simulink library "InterModuleProtocol"  (R2020b)
settings: Solver=VariableStepAuto  StartTime=0.0  StopTime=10.0  RelTol=1e-3
(part 2 of 2)

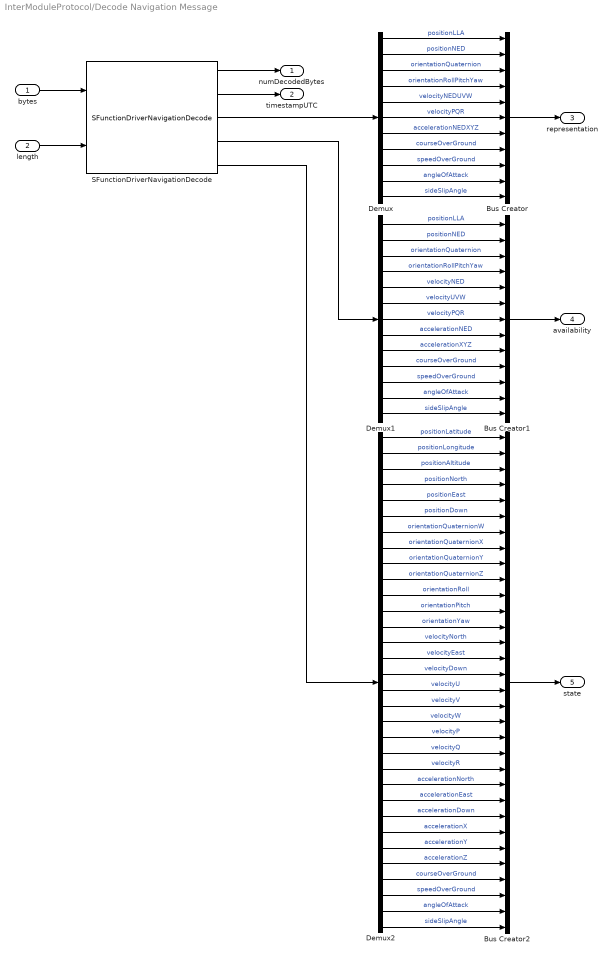
== system InterModuleProtocol/Decode Navigation Message ==
  bytes : Inport  OutDataTypeStr=uint8  PortDimensions=268
  length : Inport  Port=2  OutDataTypeStr=uint32  PortDimensions=1
  Bus Creator : BusCreator  Inputs=11
  Bus Creator1 : BusCreator  Inputs=13
  Bus Creator2 : BusCreator  Inputs=32
  Demux : Demux  Outputs=11
  Demux1 : Demux  Outputs=13
  Demux2 : Demux  Outputs=32
  SFunctionDriverNavigationDecode : S-Function  FunctionName=SFunctionDriverNavigationDecode  Parameters=SampleTime  SFunctionDeploymentMode=off  EnableBusSupport=off  mask(Legacy Function){SFunctionSpec=void OutputDriverNavigationDecode(uint8 u1[], uint32 u2, int32 y1[1], double y2[1], uint8 y3[11], uint8 y4[13], double y5[32]), SampleTime=-1, ShowSpec=off}
      mask prompts: SampleTime "Sample time (-1 for inherited):"; ShowSpec "Display function specification"
      mask help:
      | This block allows you to call the legacy functions specified by the following Legacy Code Tool definition:
      | def.SFunctionName = 'SFunctionDriverNavigationDecode';
      | def.OutputFcnSpec = 'void OutputDriverNavigationDecode(uint8 u1[], uint32 u2, int32 y1[1], double y2[1], uint8 y3[11], uint8 y4[13], double y5[32])';
      | def.StartFcnSpec = 'void CreateDriverNavigationDecode()';
      | def.TerminateFcnSpec = 'void DeleteDriverNavigationDecode()';
      | def.HeaderFiles = {'DriverNavigationDecode.h'};
      | def.SourceFiles = {'DriverNavigationDecode.cpp', 'InterModuleProtocol.cpp', 'IMPState.cpp', 'IMPStateConfiguration.cpp'};
      | def.SampleTime = 'parameterized';
      | def.Options.useTlcWithAccel = false;
      mask Help: <p>This block was generated automatically by the Legacy Code Tool. For detailed help on this tool, call<a href="matlab:legacy_code('help')"> legacy_code('help')</a>.</p>
      mask Callback ShowSpec:
      | if strcmp(get_param(gcbh, 'ShowSpec'), 'on')
      |   set_param(gcbh, 'MaskDisplay', sprintf('fprintf(''%s'');', get_param(gcbh, 'SFunctionSpec')));
      | else
      |   set_param(gcbh, 'MaskDisplay', sprintf('fprintf(''%s'');', get_param(gcbh, 'FunctionName')));
      | end
      mask Display: fprintf('SFunctionDriverNavigationDecode');
  numDecodedBytes : Outport  OutDataTypeStr=int32  PortDimensions=1  VectorParamsAs1DForOutWhenUnconnected=off
  timestampUTC : Outport  Port=2  OutDataTypeStr=double  Unit=s  PortDimensions=1  VectorParamsAs1DForOutWhenUnconnected=off
  representation : Outport  Port=3  OutDataTypeStr=uint8  PortDimensions=11  VectorParamsAs1DForOutWhenUnconnected=off
  availability : Outport  Port=4  OutDataTypeStr=uint8  PortDimensions=13  VectorParamsAs1DForOutWhenUnconnected=off
  state : Outport  Port=5  OutDataTypeStr=double  PortDimensions=32  VectorParamsAs1DForOutWhenUnconnected=off
  wires:
  SFunctionDriverNavigationDecode/1 -> numDecodedBytes/1
  SFunctionDriverNavigationDecode/2 -> timestampUTC/1
  length/1 -> SFunctionDriverNavigationDecode/2
  bytes/1 -> SFunctionDriverNavigationDecode/1
  Demux/1 -> Bus Creator/1  "positionLLA"
  Demux/2 -> Bus Creator/2  "positionNED"
  Demux/3 -> Bus Creator/3  "orientationQuaternion"
  Demux/4 -> Bus Creator/4  "orientationRollPitchYaw"
  Demux/5 -> Bus Creator/5  "velocityNEDUVW"
  Demux/6 -> Bus Creator/6  "velocityPQR"
  Demux/7 -> Bus Creator/7  "accelerationNEDXYZ"
  Demux/8 -> Bus Creator/8  "courseOverGround"
  Demux/9 -> Bus Creator/9  "speedOverGround"
  Demux/10 -> Bus Creator/10  "angleOfAttack"
  Demux/11 -> Bus Creator/11  "sideSlipAngle"
  SFunctionDriverNavigationDecode/3 -> Demux/1
  Bus Creator/1 -> representation/1
  SFunctionDriverNavigationDecode/4 -> Demux1/1
  Demux1/1 -> Bus Creator1/1  "positionLLA"
  Demux1/2 -> Bus Creator1/2  "positionNED"
  Demux1/3 -> Bus Creator1/3  "orientationQuaternion"
  Demux1/4 -> Bus Creator1/4  "orientationRollPitchYaw"
  Demux1/5 -> Bus Creator1/5  "velocityNED"
  Demux1/6 -> Bus Creator1/6  "velocityUVW"
  Demux1/7 -> Bus Creator1/7  "velocityPQR"
  Demux1/8 -> Bus Creator1/8  "accelerationNED"
  Demux1/9 -> Bus Creator1/9  "accelerationXYZ"
  Demux1/10 -> Bus Creator1/10  "courseOverGround"
  Demux1/11 -> Bus Creator1/11  "speedOverGround"
  Demux1/12 -> Bus Creator1/12  "angleOfAttack"
  Demux1/13 -> Bus Creator1/13  "sideSlipAngle"
  Bus Creator1/1 -> availability/1
  Demux2/1 -> Bus Creator2/1  "positionLatitude"
  Demux2/2 -> Bus Creator2/2  "positionLongitude"
  Demux2/3 -> Bus Creator2/3  "positionAltitude"
  Demux2/4 -> Bus Creator2/4  "positionNorth"
  Demux2/5 -> Bus Creator2/5  "positionEast"
  Demux2/6 -> Bus Creator2/6  "positionDown"
  Demux2/7 -> Bus Creator2/7  "orientationQuaternionW"
  Demux2/8 -> Bus Creator2/8  "orientationQuaternionX"
  Demux2/9 -> Bus Creator2/9  "orientationQuaternionY"
  Demux2/10 -> Bus Creator2/10  "orientationQuaternionZ"
  Demux2/11 -> Bus Creator2/11  "orientationRoll"
  Demux2/12 -> Bus Creator2/12  "orientationPitch"
  Demux2/13 -> Bus Creator2/13  "orientationYaw"
  Demux2/14 -> Bus Creator2/14  "velocityNorth"
  Demux2/15 -> Bus Creator2/15  "velocityEast"
  Demux2/16 -> Bus Creator2/16  "velocityDown"
  Demux2/17 -> Bus Creator2/17  "velocityU"
  Demux2/18 -> Bus Creator2/18  "velocityV"
  Demux2/19 -> Bus Creator2/19  "velocityW"
  Demux2/20 -> Bus Creator2/20  "velocityP"
  Demux2/21 -> Bus Creator2/21  "velocityQ"
  Demux2/22 -> Bus Creator2/22  "velocityR"
  Demux2/23 -> Bus Creator2/23  "accelerationNorth"
  Demux2/24 -> Bus Creator2/24  "accelerationEast"
  Demux2/25 -> Bus Creator2/25  "accelerationDown"
  Demux2/26 -> Bus Creator2/26  "accelerationX"
  Demux2/27 -> Bus Creator2/27  "accelerationY"
  Demux2/28 -> Bus Creator2/28  "accelerationZ"
  Demux2/29 -> Bus Creator2/29  "courseOverGround"
  Demux2/30 -> Bus Creator2/30  "speedOverGround"
  Demux2/31 -> Bus Creator2/31  "angleOfAttack"
  Demux2/32 -> Bus Creator2/32  "sideSlipAngle"
  Bus Creator2/1 -> state/1
  SFunctionDriverNavigationDecode/5 -> Demux2/1

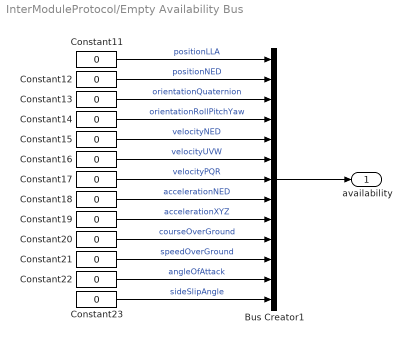
== system InterModuleProtocol/Empty Availability Bus ==
  Bus Creator1 : BusCreator  Inputs=13
  Constant{11..23} (13 alike) : Constant  Value=0  OutDataTypeStr=uint8
  availability : Outport  VectorParamsAs1DForOutWhenUnconnected=off
  wires:
  Constant21/1 -> Bus Creator1/11  "speedOverGround"
  Constant14/1 -> Bus Creator1/4  "orientationRollPitchYaw"
  Constant15/1 -> Bus Creator1/5  "velocityNED"
  Constant23/1 -> Bus Creator1/13  "sideSlipAngle"
  Bus Creator1/1 -> availability/1
  Constant12/1 -> Bus Creator1/2  "positionNED"
  Constant20/1 -> Bus Creator1/10  "courseOverGround"
  Constant16/1 -> Bus Creator1/6  "velocityUVW"
  Constant17/1 -> Bus Creator1/7  "velocityPQR"
  Constant13/1 -> Bus Creator1/3  "orientationQuaternion"
  Constant11/1 -> Bus Creator1/1  "positionLLA"
  Constant18/1 -> Bus Creator1/8  "accelerationNED"
  Constant19/1 -> Bus Creator1/9  "accelerationXYZ"
  Constant22/1 -> Bus Creator1/12  "angleOfAttack"

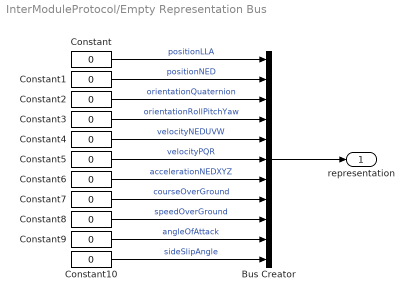
== system InterModuleProtocol/Empty Representation Bus ==
  Bus Creator : BusCreator  Inputs=11
  Constant{,1..10} (11 alike) : Constant  Value=0  OutDataTypeStr=uint8
  representation : Outport  VectorParamsAs1DForOutWhenUnconnected=off
  wires:
  Constant10/1 -> Bus Creator/11  "sideSlipAngle"
  Constant1/1 -> Bus Creator/2  "positionNED"
  Constant8/1 -> Bus Creator/9  "speedOverGround"
  Bus Creator/1 -> representation/1
  Constant9/1 -> Bus Creator/10  "angleOfAttack"
  Constant7/1 -> Bus Creator/8  "courseOverGround"
  Constant6/1 -> Bus Creator/7  "accelerationNEDXYZ"
  Constant4/1 -> Bus Creator/5  "velocityNEDUVW"
  Constant5/1 -> Bus Creator/6  "velocityPQR"
  Constant3/1 -> Bus Creator/4  "orientationRollPitchYaw"
  Constant2/1 -> Bus Creator/3  "orientationQuaternion"
  Constant/1 -> Bus Creator/1  "positionLLA"

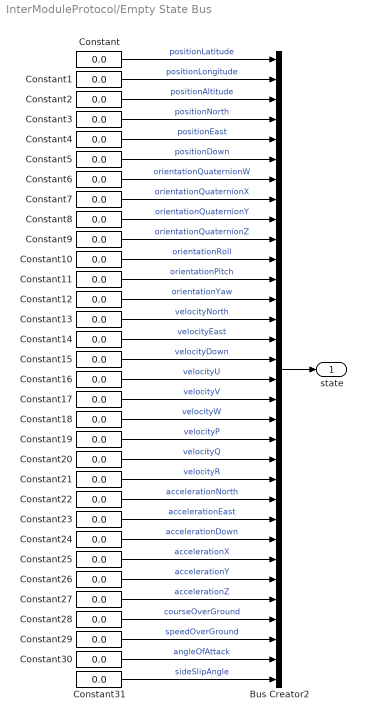
== system InterModuleProtocol/Empty State Bus ==
  Bus Creator2 : BusCreator  Inputs=32
  Constant{,1..31} (32 alike) : Constant  Value=0.0  OutDataTypeStr=double
  state : Outport  VectorParamsAs1DForOutWhenUnconnected=off
  wires:
  Constant29/1 -> Bus Creator2/30  "speedOverGround"
  Constant2/1 -> Bus Creator2/3  "positionAltitude"
  Constant8/1 -> Bus Creator2/9  "orientationQuaternionY"
  Constant17/1 -> Bus Creator2/18  "velocityV"
  Bus Creator2/1 -> state/1
  Constant25/1 -> Bus Creator2/26  "accelerationX"
  Constant1/1 -> Bus Creator2/2  "positionLongitude"
  Constant27/1 -> Bus Creator2/28  "accelerationZ"
  Constant3/1 -> Bus Creator2/4  "positionNorth"
  Constant12/1 -> Bus Creator2/13  "orientationYaw"
  Constant18/1 -> Bus Creator2/19  "velocityW"
  Constant24/1 -> Bus Creator2/25  "accelerationDown"
  Constant22/1 -> Bus Creator2/23  "accelerationNorth"
  Constant/1 -> Bus Creator2/1  "positionLatitude"
  Constant15/1 -> Bus Creator2/16  "velocityDown"
  Constant14/1 -> Bus Creator2/15  "velocityEast"
  Constant10/1 -> Bus Creator2/11  "orientationRoll"
  Constant26/1 -> Bus Creator2/27  "accelerationY"
  Constant30/1 -> Bus Creator2/31  "angleOfAttack"
  Constant6/1 -> Bus Creator2/7  "orientationQuaternionW"
  Constant13/1 -> Bus Creator2/14  "velocityNorth"
  Constant11/1 -> Bus Creator2/12  "orientationPitch"
  Constant16/1 -> Bus Creator2/17  "velocityU"
  Constant21/1 -> Bus Creator2/22  "velocityR"
  Constant19/1 -> Bus Creator2/20  "velocityP"
  Constant31/1 -> Bus Creator2/32  "sideSlipAngle"
  Constant4/1 -> Bus Creator2/5  "positionEast"
  Constant7/1 -> Bus Creator2/8  "orientationQuaternionX"
  Constant5/1 -> Bus Creator2/6  "positionDown"
  Constant9/1 -> Bus Creator2/10  "orientationQuaternionZ"
  Constant28/1 -> Bus Creator2/29  "courseOverGround"
  Constant20/1 -> Bus Creator2/21  "velocityQ"
  Constant23/1 -> Bus Creator2/24  "accelerationEast"

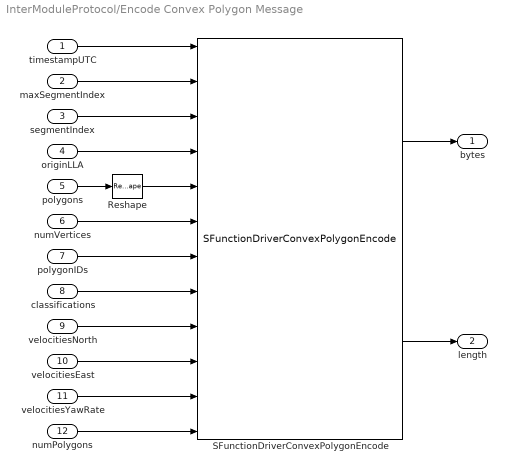
== system InterModuleProtocol/Encode Convex Polygon Message ==
  timestampUTC : Inport  OutDataTypeStr=double  Unit=s  PortDimensions=1
  maxSegmentIndex : Inport  Port=2  OutDataTypeStr=uint8  PortDimensions=1
  segmentIndex : Inport  Port=3  OutDataTypeStr=uint8  PortDimensions=1
  originLLA : Inport  Port=4  OutDataTypeStr=double  PortDimensions=3
  polygons : Inport  Port=5  OutDataTypeStr=double  Unit=m  PortDimensions=[2, 255, maxNumPolygons]
  numVertices : Inport  Port=6  OutDataTypeStr=uint8  PortDimensions=maxNumPolygons
  polygonIDs : Inport  Port=7  OutDataTypeStr=uint16  PortDimensions=maxNumPolygons
  classifications : Inport  Port=8  OutDataTypeStr=uint8  PortDimensions=maxNumPolygons
  velocitiesNorth : Inport  Port=9  OutDataTypeStr=double  Unit=m/s  PortDimensions=maxNumPolygons
  velocitiesEast : Inport  Port=10  OutDataTypeStr=double  Unit=m/s  PortDimensions=maxNumPolygons
  velocitiesYawRate : Inport  Port=11  OutDataTypeStr=double  Unit=rad/s  PortDimensions=maxNumPolygons
  numPolygons : Inport  Port=12  OutDataTypeStr=uint16  PortDimensions=1
  Reshape : Reshape  OutputDimensionality=Customize  OutputDimensions=[2*255*maxNumPolygons,1]
  SFunctionDriverConvexPolygonEncode : S-Function  FunctionName=SFunctionDriverConvexPolygonEncode  Parameters=SParameter1, SParameter2, SampleTime  SFunctionDeploymentMode=off  EnableBusSupport=off  mask(Legacy Function){SFunctionSpec=void OutputDriverConvexPolygonEncode(uint8 y1[p1], uint32 y2[1], uint32 p1, double u1, uint8 u2, uint8 u3, double u4[3], double u5[2*255*p2], uint16 p2, uint8 u6[p2], uint8 u7[p2], uint8 u8[p2], double u9[p2], double u10[p2], double u11[p2], uint16 u12), SParameter1=uint32(reshape(outBufferSize, [1 1])), SParameter2=uint16(reshape(maxNumPolygons, [1 1])), SampleTime=-1, ShowSpec=off}
      mask prompts: SParameter1 "P1:"; SParameter2 "P2:"; SampleTime "Sample time (-1 for inherited):"; ShowSpec "Display function specification"
      mask help:
      | This block allows you to call the legacy functions specified by the following Legacy Code Tool definition:
      | def.SFunctionName = 'SFunctionDriverConvexPolygonEncode';
      | def.OutputFcnSpec = 'void OutputDriverConvexPolygonEncode(uint8 y1[p1], uint32 y2[1], uint32 p1, double u1, uint8 u2, uint8 u3, double u4[3], double u5[2*255*p2], uint16 p2, uint8 u6[p2], uint8 u7[p2], uint8 u8[p2], double u9[p2], double u10[p2], double u11[p2], uint16 u12)';
      | def.StartFcnSpec = 'void CreateDriverConvexPolygonEncode()';
      | def.TerminateFcnSpec = 'void DeleteDriverConvexPolygonEncode()';
      | def.HeaderFiles = {'DriverConvexPolygonEncode.h'};
      | def.SourceFiles = {'DriverConvexPolygonEncode.cpp', 'InterModuleProtocol.cpp', 'IMPState.cpp', 'IMPConvexPolygon.cpp', 'IMPStateConfiguration.cpp'};
      | def.SampleTime = 'parameterized';
      | def.Options.useTlcWithAccel = false;
      mask Help: <p>This block was generated automatically by the Legacy Code Tool. For detailed help on this tool, call<a href="matlab:legacy_code('help')"> legacy_code('help')</a>.</p>
      mask Callback ShowSpec:
      | if strcmp(get_param(gcbh, 'ShowSpec'), 'on')
      |   set_param(gcbh, 'MaskDisplay', sprintf('fprintf(''%s'');', get_param(gcbh, 'SFunctionSpec')));
      | else
      |   set_param(gcbh, 'MaskDisplay', sprintf('fprintf(''%s'');', get_param(gcbh, 'FunctionName')));
      | end
      mask Display: fprintf('SFunctionDriverConvexPolygonEncode');
  bytes : Outport  OutDataTypeStr=uint8  PortDimensions=outBufferSize  VectorParamsAs1DForOutWhenUnconnected=off
  length : Outport  Port=2  OutDataTypeStr=uint32  PortDimensions=1  VectorParamsAs1DForOutWhenUnconnected=off
  wires:
  polygons/1 -> Reshape/1
  SFunctionDriverConvexPolygonEncode/1 -> bytes/1
  SFunctionDriverConvexPolygonEncode/2 -> length/1
  timestampUTC/1 -> SFunctionDriverConvexPolygonEncode/1
  maxSegmentIndex/1 -> SFunctionDriverConvexPolygonEncode/2
  segmentIndex/1 -> SFunctionDriverConvexPolygonEncode/3
  originLLA/1 -> SFunctionDriverConvexPolygonEncode/4
  Reshape/1 -> SFunctionDriverConvexPolygonEncode/5
  numVertices/1 -> SFunctionDriverConvexPolygonEncode/6
  polygonIDs/1 -> SFunctionDriverConvexPolygonEncode/7
  numPolygons/1 -> SFunctionDriverConvexPolygonEncode/12
  classifications/1 -> SFunctionDriverConvexPolygonEncode/8
  velocitiesNorth/1 -> SFunctionDriverConvexPolygonEncode/9
  velocitiesEast/1 -> SFunctionDriverConvexPolygonEncode/10
  velocitiesYawRate/1 -> SFunctionDriverConvexPolygonEncode/11

== system InterModuleProtocol/Encode Guidance Message ==
  timestampUTC : Inport  OutDataTypeStr=double  Unit=s  PortDimensions=1
  representation : Inport  Port=2  OutDataTypeStr=uint8  PortDimensions=11
  availability : Inport  Port=3  OutDataTypeStr=uint8  PortDimensions=13
  state : Inport  Port=4  OutDataTypeStr=double  PortDimensions=32
  SFunctionDriverGuidanceEncode : S-Function  FunctionName=SFunctionDriverGuidanceEncode  Parameters=SParameter1, SampleTime  SFunctionDeploymentMode=off  EnableBusSupport=off  mask(Legacy Function){SFunctionSpec=void OutputDriverGuidanceEncode(uint8 y1[p1], uint32 y2[1], uint32 p1, double u1, uint8 u2[11], uint8 u3[13], double u4[32]), SParameter1=uint32(reshape(outputBufferSize, [1 1])), SampleTime=-1, ShowSpec=off}
      mask prompts: SParameter1 "P1:"; SampleTime "Sample time (-1 for inherited):"; ShowSpec "Display function specification"
      mask help:
      | This block allows you to call the legacy functions specified by the following Legacy Code Tool definition:
      | def.SFunctionName = 'SFunctionDriverGuidanceEncode';
      | def.OutputFcnSpec = 'void OutputDriverGuidanceEncode(uint8 y1[p1], uint32 y2[1], uint32 p1, double u1, uint8 u2[11], uint8 u3[13], double u4[32])';
      | def.StartFcnSpec = 'void CreateDriverGuidanceEncode()';
      | def.TerminateFcnSpec = 'void DeleteDriverGuidanceEncode()';
      | def.HeaderFiles = {'DriverGuidanceEncode.h'};
      | def.SourceFiles = {'DriverGuidanceEncode.cpp', 'InterModuleProtocol.cpp', 'IMPConvexPolygon.cpp', 'IMPState.cpp', 'IMPStateConfiguration.cpp'};
      | def.SampleTime = 'parameterized';
      | def.Options.useTlcWithAccel = false;
      mask Help: <p>This block was generated automatically by the Legacy Code Tool. For detailed help on this tool, call<a href="matlab:legacy_code('help')"> legacy_code('help')</a>.</p>
      mask Callback ShowSpec:
      | if strcmp(get_param(gcbh, 'ShowSpec'), 'on')
      |   set_param(gcbh, 'MaskDisplay', sprintf('fprintf(''%s'');', get_param(gcbh, 'SFunctionSpec')));
      | else
      |   set_param(gcbh, 'MaskDisplay', sprintf('fprintf(''%s'');', get_param(gcbh, 'FunctionName')));
      | end
      mask Display: fprintf('SFunctionDriverGuidanceEncode');
  bytes : Outport  OutDataTypeStr=uint8  PortDimensions=outputBufferSize  VectorParamsAs1DForOutWhenUnconnected=off
  length : Outport  Port=2  OutDataTypeStr=uint32  PortDimensions=1  VectorParamsAs1DForOutWhenUnconnected=off
  wires:
  timestampUTC/1 -> SFunctionDriverGuidanceEncode/1
  representation/1 -> SFunctionDriverGuidanceEncode/2
  availability/1 -> SFunctionDriverGuidanceEncode/3
  state/1 -> SFunctionDriverGuidanceEncode/4
  SFunctionDriverGuidanceEncode/1 -> bytes/1
  SFunctionDriverGuidanceEncode/2 -> length/1

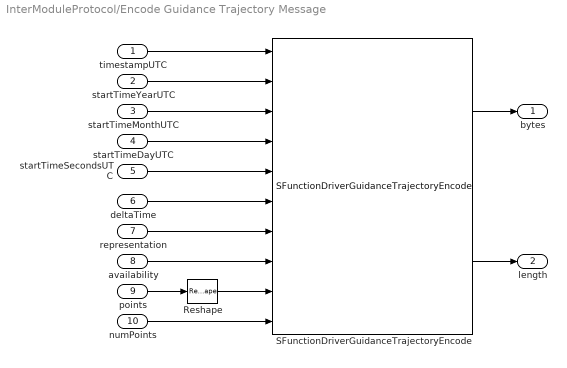
== system InterModuleProtocol/Encode Guidance Trajectory Message ==
  timestampUTC : Inport  OutDataTypeStr=double  Unit=s  PortDimensions=1
  startTimeYearUTC : Inport  Port=2  OutDataTypeStr=int32  PortDimensions=1
  startTimeMonthUTC : Inport  Port=3  OutDataTypeStr=int32  PortDimensions=1
  startTimeDayUTC : Inport  Port=4  OutDataTypeStr=int32  PortDimensions=1
  startTimeSecondsUTC : Inport  Port=5  OutDataTypeStr=double  Unit=s  PortDimensions=1
  deltaTime : Inport  Port=6  OutDataTypeStr=double  Unit=s  PortDimensions=1
  representation : Inport  Port=7  OutDataTypeStr=uint8  PortDimensions=11
  availability : Inport  Port=8  OutDataTypeStr=uint8  PortDimensions=13
  points : Inport  Port=9  OutDataTypeStr=double  PortDimensions=[32, maxNumPoints]
  numPoints : Inport  Port=10  OutDataTypeStr=uint32  PortDimensions=1
  Reshape : Reshape  OutputDimensionality=Customize  OutputDimensions=[32*maxNumPoints,1]
  SFunctionDriverGuidanceTrajectoryEncode : S-Function  FunctionName=SFunctionDriverGuidanceTrajectoryEncode  Parameters=SParameter1, SParameter2, SampleTime  SFunctionDeploymentMode=off  EnableBusSupport=off  mask(Legacy Function){SFunctionSpec=void OutputDriverGuidanceTrajectoryEncode(uint8 y1[p1], uint32 y2[1], uint32 p1, double u1, int32 u2, int32 u3, int32 u4, double u5, double u6, uint8 u7[11], uint8 u8[13], double u9[32*p2], uint32 p2, uint32 u10), SParameter1=uint32(reshape(outputBufferSize, [1 1])), SParameter2=uint32(reshape(maxNumPoints, [1 1])), SampleTime=-1, ShowSpec=off}
      mask prompts: SParameter1 "P1:"; SParameter2 "P2:"; SampleTime "Sample time (-1 for inherited):"; ShowSpec "Display function specification"
      mask help:
      | This block allows you to call the legacy functions specified by the following Legacy Code Tool definition:
      | def.SFunctionName = 'SFunctionDriverGuidanceTrajectoryEncode';
      | def.OutputFcnSpec = 'void OutputDriverGuidanceTrajectoryEncode(uint8 y1[p1], uint32 y2[1], uint32 p1, double u1, int32 u2, int32 u3, int32 u4, double u5, double u6, uint8 u7[11], uint8 u8[13], double u9[32*p2], uint32 p2, uint32 u10)';
      | def.StartFcnSpec = 'void CreateDriverGuidanceTrajectoryEncode()';
      | def.TerminateFcnSpec = 'void DeleteDriverGuidanceTrajectoryEncode()';
      | def.HeaderFiles = {'DriverGuidanceTrajectoryEncode.h'};
      | def.SourceFiles = {'DriverGuidanceTrajectoryEncode.cpp', 'InterModuleProtocol.cpp', 'IMPConvexPolygon.cpp', 'IMPState.cpp', 'IMPStateConfiguration.cpp'};
      | def.IncPaths = {'..\..\source\InterModuleProtocol'};
      | def.SrcPaths = {'..\..\source\InterModuleProtocol'};
      | def.SampleTime = 'parameterized';
      | def.Options.useTlcWithAccel = false;
      mask Help: <p>This block was generated automatically by the Legacy Code Tool. For detailed help on this tool, call<a href="matlab:legacy_code('help')"> legacy_code('help')</a>.</p>
      mask Callback ShowSpec:
      | if strcmp(get_param(gcbh, 'ShowSpec'), 'on')
      |   set_param(gcbh, 'MaskDisplay', sprintf('fprintf(''%s'');', get_param(gcbh, 'SFunctionSpec')));
      | else
      |   set_param(gcbh, 'MaskDisplay', sprintf('fprintf(''%s'');', get_param(gcbh, 'FunctionName')));
      | end
      mask Display: fprintf('SFunctionDriverGuidanceTrajectoryEncode');
  bytes : Outport  OutDataTypeStr=uint8  VectorParamsAs1DForOutWhenUnconnected=off
  length : Outport  Port=2  OutDataTypeStr=uint32  PortDimensions=1  VectorParamsAs1DForOutWhenUnconnected=off
  wires:
  SFunctionDriverGuidanceTrajectoryEncode/1 -> bytes/1
  timestampUTC/1 -> SFunctionDriverGuidanceTrajectoryEncode/1
  deltaTime/1 -> SFunctionDriverGuidanceTrajectoryEncode/6
  availability/1 -> SFunctionDriverGuidanceTrajectoryEncode/8
  SFunctionDriverGuidanceTrajectoryEncode/2 -> length/1
  points/1 -> Reshape/1
  representation/1 -> SFunctionDriverGuidanceTrajectoryEncode/7
  startTimeYearUTC/1 -> SFunctionDriverGuidanceTrajectoryEncode/2
  startTimeMonthUTC/1 -> SFunctionDriverGuidanceTrajectoryEncode/3
  startTimeDayUTC/1 -> SFunctionDriverGuidanceTrajectoryEncode/4
  startTimeSecondsUTC/1 -> SFunctionDriverGuidanceTrajectoryEncode/5
  Reshape/1 -> SFunctionDriverGuidanceTrajectoryEncode/9
  numPoints/1 -> SFunctionDriverGuidanceTrajectoryEncode/10

== system InterModuleProtocol/Encode Info Request Message ==
  timestampUTC : Inport  OutDataTypeStr=double  Unit=s  PortDimensions=1
  SFunctionDriverInfoRequestEncode : S-Function  FunctionName=SFunctionDriverInfoRequestEncode  Parameters=SParameter1, SampleTime  SFunctionDeploymentMode=off  EnableBusSupport=off  mask(Legacy Function){SFunctionSpec=void OutputDriverInfoRequestEncode(uint8 y1[p1], uint32 y2[1], uint32 p1, double u1), SParameter1=uint32(reshape(outputBufferSize, [1 1])), SampleTime=-1, ShowSpec=on}
      mask prompts: SParameter1 "P1:"; SampleTime "Sample time (-1 for inherited):"; ShowSpec "Display function specification"
      mask help:
      | This block allows you to call the legacy functions specified by the following Legacy Code Tool definition:
      | def.SFunctionName = 'SFunctionDriverInfoRequestEncode';
      | def.OutputFcnSpec = 'void OutputDriverInfoRequestEncode(uint8 y1[p1], uint32 y2[1], uint32 p1, double u1)';
      | def.StartFcnSpec = 'void CreateDriverInfoRequestEncode()';
      | def.TerminateFcnSpec = 'void DeleteDriverInfoRequestEncode()';
      | def.HeaderFiles = {'DriverInfoRequestEncode.h'};
      | def.SourceFiles = {'DriverInfoRequestEncode.cpp', 'InterModuleProtocol.cpp', 'IMPConvexPolygon.cpp', 'IMPState.cpp', 'IMPStateConfiguration.cpp'};
      | def.SampleTime = 'parameterized';
      | def.Options.useTlcWithAccel = false;
      mask Help: <p>This block was generated automatically by the Legacy Code Tool. For detailed help on this tool, call<a href="matlab:legacy_code('help')"> legacy_code('help')</a>.</p>
      mask Callback ShowSpec:
      | if strcmp(get_param(gcbh, 'ShowSpec'), 'on')
      |   set_param(gcbh, 'MaskDisplay', sprintf('fprintf(''%s'');', get_param(gcbh, 'SFunctionSpec')));
      | else
      |   set_param(gcbh, 'MaskDisplay', sprintf('fprintf(''%s'');', get_param(gcbh, 'FunctionName')));
      | end
      mask Display: fprintf('void OutputDriverInfoRequestEncode(uint8 y1[p1], uint32 y2[1], uint32 p1, double u1)');
  bytes : Outport  OutDataTypeStr=uint8  PortDimensions=outputBufferSize  VectorParamsAs1DForOutWhenUnconnected=off
  length : Outport  Port=2  OutDataTypeStr=uint32  PortDimensions=1  VectorParamsAs1DForOutWhenUnconnected=off
  wires:
  timestampUTC/1 -> SFunctionDriverInfoRequestEncode/1
  SFunctionDriverInfoRequestEncode/2 -> length/1
  SFunctionDriverInfoRequestEncode/1 -> bytes/1

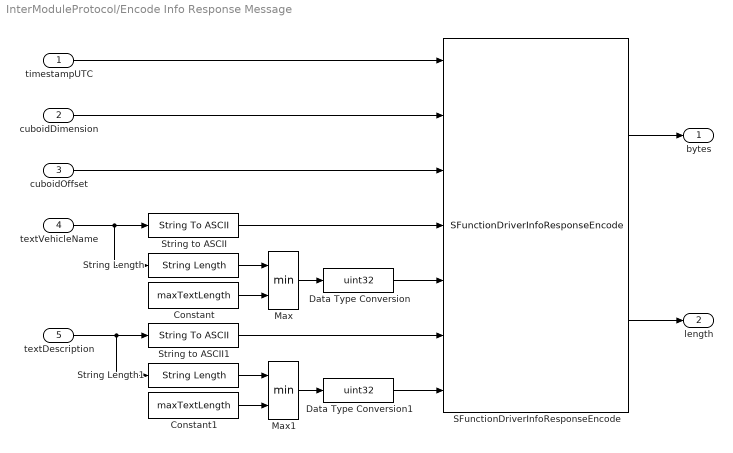
== system InterModuleProtocol/Encode Info Response Message ==
  timestampUTC : Inport  OutDataTypeStr=double  Unit=s  PortDimensions=1
  cuboidDimension : Inport  Port=2  OutDataTypeStr=double  Unit=m  PortDimensions=3
  cuboidOffset : Inport  Port=3  OutDataTypeStr=double  Unit=m  PortDimensions=3
  textVehicleName : Inport  Port=4
  textDescription : Inport  Port=5
  Constant : Constant  Value=maxTextLength
  Constant1 : Constant  Value=maxTextLength
  Data Type Conversion : DataTypeConversion  OutDataTypeStr=uint32
  Data Type Conversion1 : DataTypeConversion  OutDataTypeStr=uint32
  Max : MinMax  Inputs=2
  Max1 : MinMax  Inputs=2
  SFunctionDriverInfoResponseEncode : S-Function  FunctionName=SFunctionDriverInfoResponseEncode  Parameters=SParameter1, SParameter2, SampleTime  SFunctionDeploymentMode=off  EnableBusSupport=off  mask(Legacy Function){SFunctionSpec=void OutputDriverInfoResponseEncode(uint8 y1[p1], uint32 y2[1], uint32 p1, double u1, double u2[3], double u3[3], uint8 u4[p2], uint32 u5, uint8 u6[p2], uint32 u7, uint32 p2), SParameter1=uint32(reshape(outputBufferSize, [1 1])), SParameter2=uint32(reshape(maxTextLength, [1 1])), SampleTime=-1, ShowSpec=off}
      mask prompts: SParameter1 "P1:"; SParameter2 "P2:"; SampleTime "Sample time (-1 for inherited):"; ShowSpec "Display function specification"
      mask help:
      | This block allows you to call the legacy functions specified by the following Legacy Code Tool definition:
      | def.SFunctionName = 'SFunctionDriverInfoResponseEncode';
      | def.OutputFcnSpec = 'void OutputDriverInfoResponseEncode(uint8 y1[p1], uint32 y2[1], uint32 p1, double u1, double u2[3], double u3[3], uint8 u4[p2], uint32 u5, uint8 u6[p2], uint32 u7, uint32 p2)';
      | def.StartFcnSpec = 'void CreateDriverInfoResponseEncode()';
      | def.TerminateFcnSpec = 'void DeleteDriverInfoResponseEncode()';
      | def.HeaderFiles = {'DriverInfoResponseEncode.h'};
      | def.SourceFiles = {'DriverInfoResponseEncode.cpp', 'InterModuleProtocol.cpp', 'IMPState.cpp', 'IMPStateConfiguration.cpp'};
      | def.SampleTime = 'parameterized';
      | def.Options.useTlcWithAccel = false;
      mask Help: <p>This block was generated automatically by the Legacy Code Tool. For detailed help on this tool, call<a href="matlab:legacy_code('help')"> legacy_code('help')</a>.</p>
      mask Callback ShowSpec:
      | if strcmp(get_param(gcbh, 'ShowSpec'), 'on')
      |   set_param(gcbh, 'MaskDisplay', sprintf('fprintf(''%s'');', get_param(gcbh, 'SFunctionSpec')));
      | else
      |   set_param(gcbh, 'MaskDisplay', sprintf('fprintf(''%s'');', get_param(gcbh, 'FunctionName')));
      | end
      mask Display: fprintf('SFunctionDriverInfoResponseEncode');
  String Length : StringLength
  String Length1 : StringLength
  String to ASCII : StringToASCII  OutputVectorSize=maxTextLength
  String to ASCII1 : StringToASCII  OutputVectorSize=maxTextLength
  bytes : Outport  OutDataTypeStr=uint8  PortDimensions=outputBufferSize  VectorParamsAs1DForOutWhenUnconnected=off
  length : Outport  Port=2  OutDataTypeStr=uint32  PortDimensions=1  VectorParamsAs1DForOutWhenUnconnected=off
  wires:
  SFunctionDriverInfoResponseEncode/1 -> bytes/1
  cuboidOffset/1 -> SFunctionDriverInfoResponseEncode/3
  textDescription/1 -> String Length1/1, String to ASCII1/1
  cuboidDimension/1 -> SFunctionDriverInfoResponseEncode/2
  timestampUTC/1 -> SFunctionDriverInfoResponseEncode/1
  SFunctionDriverInfoResponseEncode/2 -> length/1
  textVehicleName/1 -> String Length/1, String to ASCII/1
  String to ASCII/1 -> SFunctionDriverInfoResponseEncode/4
  String to ASCII1/1 -> SFunctionDriverInfoResponseEncode/6
  Max/1 -> Data Type Conversion/1
  Constant/1 -> Max/2
  String Length/1 -> Max/1
  Data Type Conversion/1 -> SFunctionDriverInfoResponseEncode/5
  String Length1/1 -> Max1/1
  Constant1/1 -> Max1/2
  Max1/1 -> Data Type Conversion1/1
  Data Type Conversion1/1 -> SFunctionDriverInfoResponseEncode/7

== system InterModuleProtocol/Encode Log Message ==
  timestampUTC : Inport  OutDataTypeStr=double  Unit=s  PortDimensions=1
  color : Inport  Port=2  OutDataTypeStr=uint8  PortDimensions=3
  text : Inport  Port=3
  Constant : Constant  Value=maxTextLength
  Data Type Conversion : DataTypeConversion  OutDataTypeStr=uint32
  Max : MinMax  Inputs=2
  SFunctionDriverLogEncode : S-Function  FunctionName=SFunctionDriverLogEncode  Parameters=SParameter1, SParameter2, SampleTime  SFunctionDeploymentMode=off  EnableBusSupport=off  mask(Legacy Function){SFunctionSpec=void OutputDriverLogEncode(uint8 y1[p1], uint32 y2[1], uint32 p1, double u1, uint8 u2[3], uint8 u3[p2], uint32 p2, uint32 u4), SParameter1=uint32(reshape(outputBufferSize, [1 1])), SParameter2=uint32(reshape(maxTextLength, [1 1])), SampleTime=-1, ShowSpec=off}
      mask prompts: SParameter1 "P1:"; SParameter2 "P2:"; SampleTime "Sample time (-1 for inherited):"; ShowSpec "Display function specification"
      mask help:
      | This block allows you to call the legacy functions specified by the following Legacy Code Tool definition:
      | def.SFunctionName = 'SFunctionDriverLogEncode';
      | def.OutputFcnSpec = 'void OutputDriverLogEncode(uint8 y1[p1], uint32 y2[1], uint32 p1, double u1, uint8 u2[3], uint8 u3[p2], uint32 p2, uint32 u4)';
      | def.StartFcnSpec = 'void CreateDriverLogEncode()';
      | def.TerminateFcnSpec = 'void DeleteDriverLogEncode()';
      | def.HeaderFiles = {'DriverLogEncode.h'};
      | def.SourceFiles = {'DriverLogEncode.cpp', 'InterModuleProtocol.cpp', 'IMPState.cpp', 'IMPStateConfiguration.cpp'};
      | def.SampleTime = 'parameterized';
      | def.Options.useTlcWithAccel = false;
      mask Help: <p>This block was generated automatically by the Legacy Code Tool. For detailed help on this tool, call<a href="matlab:legacy_code('help')"> legacy_code('help')</a>.</p>
      mask Callback ShowSpec:
      | if strcmp(get_param(gcbh, 'ShowSpec'), 'on')
      |   set_param(gcbh, 'MaskDisplay', sprintf('fprintf(''%s'');', get_param(gcbh, 'SFunctionSpec')));
      | else
      |   set_param(gcbh, 'MaskDisplay', sprintf('fprintf(''%s'');', get_param(gcbh, 'FunctionName')));
      | end
      mask Display: fprintf('SFunctionDriverLogEncode');
  String Length : StringLength
  String to ASCII : StringToASCII  OutputVectorSize=maxTextLength
  bytes : Outport  OutDataTypeStr=uint8  PortDimensions=outputBufferSize  VectorParamsAs1DForOutWhenUnconnected=off
  length : Outport  Port=2  OutDataTypeStr=uint32  PortDimensions=1  VectorParamsAs1DForOutWhenUnconnected=off
  wires:
  text/1 -> String Length/1, String to ASCII/1
  SFunctionDriverLogEncode/1 -> bytes/1
  SFunctionDriverLogEncode/2 -> length/1
  timestampUTC/1 -> SFunctionDriverLogEncode/1
  color/1 -> SFunctionDriverLogEncode/2
  String to ASCII/1 -> SFunctionDriverLogEncode/3
  String Length/1 -> Max/1
  Data Type Conversion/1 -> SFunctionDriverLogEncode/4
  Constant/1 -> Max/2
  Max/1 -> Data Type Conversion/1

== system InterModuleProtocol/Encode Navigation Message ==
  timestampUTC : Inport  OutDataTypeStr=double  Unit=s  PortDimensions=1
  representation : Inport  Port=2  OutDataTypeStr=uint8  PortDimensions=11
  availability : Inport  Port=3  OutDataTypeStr=uint8  PortDimensions=13
  state : Inport  Port=4  OutDataTypeStr=double  PortDimensions=32
  SFunctionDriverNavigationEncode : S-Function  FunctionName=SFunctionDriverNavigationEncode  Parameters=SParameter1, SampleTime  SFunctionDeploymentMode=off  EnableBusSupport=off  mask(Legacy Function){SFunctionSpec=void OutputDriverNavigationEncode(uint8 y1[p1], uint32 y2[1], uint32 p1, double u1, uint8 u2[11], uint8 u3[13], double u4[32]), SParameter1=uint32(reshape(outputBufferSize, [1 1])), SampleTime=-1, ShowSpec=off}
      mask prompts: SParameter1 "P1:"; SampleTime "Sample time (-1 for inherited):"; ShowSpec "Display function specification"
      mask help:
      | This block allows you to call the legacy functions specified by the following Legacy Code Tool definition:
      | def.SFunctionName = 'SFunctionDriverNavigationEncode';
      | def.OutputFcnSpec = 'void OutputDriverNavigationEncode(uint8 y1[p1], uint32 y2[1], uint32 p1, double u1, uint8 u2[11], uint8 u3[13], double u4[32])';
      | def.StartFcnSpec = 'void CreateDriverNavigationEncode()';
      | def.TerminateFcnSpec = 'void DeleteDriverNavigationEncode()';
      | def.HeaderFiles = {'DriverNavigationEncode.h'};
      | def.SourceFiles = {'DriverNavigationEncode.cpp', 'InterModuleProtocol.cpp', 'IMPConvexPolygon.cpp', 'IMPState.cpp', 'IMPStateConfiguration.cpp'};
      | def.SampleTime = 'parameterized';
      | def.Options.useTlcWithAccel = false;
      mask Help: <p>This block was generated automatically by the Legacy Code Tool. For detailed help on this tool, call<a href="matlab:legacy_code('help')"> legacy_code('help')</a>.</p>
      mask Callback ShowSpec:
      | if strcmp(get_param(gcbh, 'ShowSpec'), 'on')
      |   set_param(gcbh, 'MaskDisplay', sprintf('fprintf(''%s'');', get_param(gcbh, 'SFunctionSpec')));
      | else
      |   set_param(gcbh, 'MaskDisplay', sprintf('fprintf(''%s'');', get_param(gcbh, 'FunctionName')));
      | end
      mask Display: fprintf('SFunctionDriverNavigationEncode');
  bytes : Outport  OutDataTypeStr=uint8  PortDimensions=outputBufferSize  VectorParamsAs1DForOutWhenUnconnected=off
  length : Outport  Port=2  OutDataTypeStr=uint32  PortDimensions=1  VectorParamsAs1DForOutWhenUnconnected=off
  wires:
  SFunctionDriverNavigationEncode/1 -> bytes/1
  state/1 -> SFunctionDriverNavigationEncode/4
  timestampUTC/1 -> SFunctionDriverNavigationEncode/1
  representation/1 -> SFunctionDriverNavigationEncode/2
  availability/1 -> SFunctionDriverNavigationEncode/3
  SFunctionDriverNavigationEncode/2 -> length/1
